simulink model "PathFollowing"  (R2020b)
settings: Solver=FixedStepAuto  StartTime=0.0  StopTime=inf  FixedStep=0.1  RelTol=1e-3
InitFcn:
  | InitParam;
  | SetWaypoints;
StopFcn:
  | plotTrack;
values from neighbouring files (symbols this model uses):
  P0 = [0,0]    [SetWaypoints.m]
  Waypoints = [0 30; 30 30; 30 -30; -30 -30; -30 0; -5 0]    [SetWaypoints.m]
  WPNum = size(Waypoints,1)    [SetWaypoints.m]
  Yaw0 = 70    [SetWaypoints.m]
libraries: vrlib x2, pid_lib x1
settings Model: Creator=53549  LastModifiedBy=53549
settings DataIOCC: ReturnWorkspaceOutputs=off
settings DebuggingCC: ArithmeticOperatorsInVariantConditions=warning
settings SFSimCC: SimUseLocalCustomCode=off  CustomCodeUndefinedFunction=UseInterfaceOnly
settings RTWCC: RTWUseLocalCustomCode=off
settings CodeAppCC: StateflowObjectComments=on

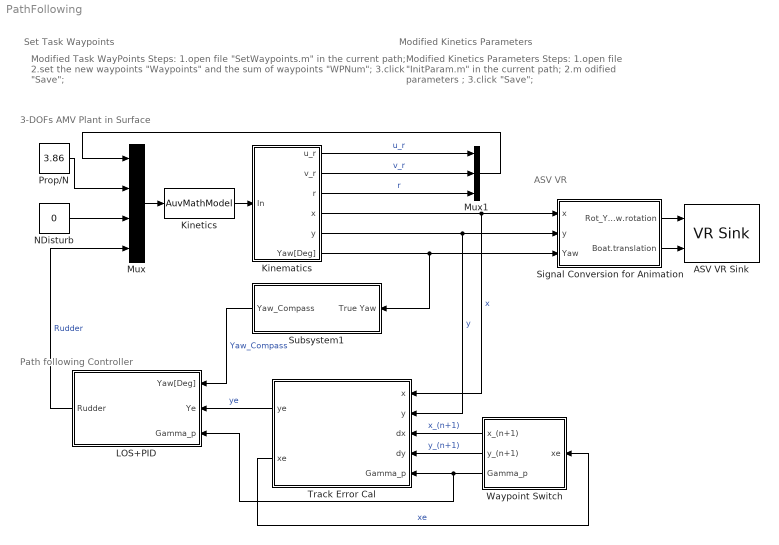
== system PathFollowing ==
  note: ASV VR
  note: Set Task Waypoints
  note: Modified Task WayPoints Steps:
      | 1.open file "SetWaypoints.m" in the current path;
      | 2.set the new waypoints "Waypoints" and the sum of waypoints "WPNum";
      | 3.click "Save";
  note: Path following Controller
  note: 3-DOFs AMV Plant in Surface
  note: Modified Kinetics Parameters
  note: Modified Kinetics Parameters Steps:
      | 1.open file "InitParam.m" in the current path;
      | 2.m odified parameters ;
      | 3.click "Save";
  ASV VR Sink : vrlib/VR Sink  InstantiateOnLoad=on  SampleTime=0.1  ViewEnable=on  RemoteChange=off  RemoteView=off  FieldsWritten=Boat.rotation.4.1.1.double#Boat.translation.3.1.1.double  WorldFileName=ASV.x3d  WorldDescription=ASV Simulation Animation  AutoView=off  VideoDimensions=[]  AllowVariableSize=off  FigureProperties="{'Position', 'Name', 'Viewpoint', 'CameraBound', 'CameraDirection', 'CameraPosition', 'CameraUpVector', 'ZoomFactor', 'Antialiasing', 'Headlight', 'Lighting', 'NavPanel', 'Sound', 'StatusBar', 'Stereo3D', 'Stereo3DCameraOffset', 'Stereo3DHIT', 'ToolBar', 'Textures', 'Transparency', 'Triad', 'Wireframe', 'NavZones', 'NavMode', 'NavSpeed', 'CaptureFileFormat', 'CaptureFileName', 'Record2DCompressMethod', 'Record2DCompressQuality', 'Record2D', 'Record2DFileName', 'Record2DFPS'; [5.0000000000000000e+00   9.2000000000000000e+01   5.7600000000000000e+02   3.5000000000000000e+02], 'ASV Simulation Animation', 'OverView_100m', 'on', [0.0000000000000000e+00   0.0000000000000000e+00  -1.0000000000000000e+00], [0.0000000000000000e+00   0.0000000000000000e+00  -6.0000000000000000e+00], [0.0000000000000000e+00   1.0000000000000000e+00   0.0000000000000000e+00], [1.0000000000000000e+00], 'on', 'on', 'on', 'halfbar', 'on', 'on', 'off', [1.0000000149011612e-01], [0.0000000000000000e+00], 'on', 'on', 'on', 'none', 'off', 'off', 'fly', 'normal', 'tif', '%f_anim_%n.tif', 'auto', [7.5000000000000000e+01], 'off', '%f_anim_%n.avi', 'auto'}"
  "Kinematics " : Subsystem  mask{yawInit=Yaw0, u0=0.4, flowDir=45, flowVel=0.2}
      mask prompts: yawInit "Initial yaw [Deg]"; u0 "Initial velocity [m/s]"; flowDir "Flow direction [Deg]"; flowVel "Flow velocity [m/s]"
      mask DialogControl DescGroupVar Prompt: Kinematics
      mask DialogControl DescTextVar Prompt: Set kinematics information: ASV initial state, flow disturance, etc
      mask DialogControl ParameterGroupVar Prompt: Initial state
      mask DialogControl Container3 Prompt: Flow
  Kinetics : MATLABFcn  MATLABFcn=AuvMathModel  OutputDimensions=3  OutputSignalType=real
  LOS+PID : Subsystem  mask{kp=1, ki=0, kd=1.5, losAlg=ALOS, klos=3, KIlos=0.04}
      mask prompts: losAlg "Guidance Form"
      mask TypeOptions losAlg: LOS | ALOS
      mask DialogControl DescGroupVar Prompt: Path following control
      mask DialogControl DescTextVar Prompt: Please select the guidance law and set the parameters of heading autopilot and line of sight guidance.
      mask DialogControl ParameterGroupVar Prompt: Heading  Autopilot
      mask DialogControl Container3 Prompt: Guidance
  Mux : Mux
  Mux1 : Mux  Inputs=3
  NDisturb : Constant  Value=0
  Prop/N : Constant  Value=3.86
  Signal Conversion for Animation : Subsystem
  Subsystem1 : Subsystem
  Track Error Cal : MATLAB Function  TreatAsAtomicUnit=on
  Waypoint Switch : Subsystem  mask{WP=Waypoints, WPNum=WPNum}
      mask prompts: WP "Waypoints"; WPNum "Waypoints Sum"
      mask DialogControl DescGroupVar Prompt: Task Waypoints
      mask DialogControl DescTextVar Prompt: Please set waypoints and the sum.
  wires:
  Kinetics/1 -> "Kinematics "/1(In)
  Mux/1 -> Kinetics/1
  "Kinematics "/6(Yaw[Deg]) -> Subsystem1/1(True Yaw), Signal Conversion for Animation/3(Yaw)
  "Kinematics "/1(u_r) -> Mux1/1  "u_r"
  "Kinematics "/2(v_r) -> Mux1/2  "v_r"
  "Kinematics "/3(r) -> Mux1/3  "r"
  Mux1/1 -> Mux/1
  Prop/N/1 -> Mux/2
  "Kinematics "/4(x) -> Track Error Cal/1(x), Signal Conversion for Animation/1(x)  "x"
  "Kinematics "/5(y) -> Track Error Cal/2(y), Signal Conversion for Animation/2(y)  "y"
  LOS+PID/1(Rudder) -> Mux/4  "Rudder"
  NDisturb/1 -> Mux/3
  Track Error Cal/1(ye) -> LOS+PID/2(Ye)  "ye"
  Track Error Cal/2(xe) -> Waypoint Switch/1(xe)  "xe"
  Waypoint Switch/1(x_(n+1)) -> Track Error Cal/3(dx)  "x_(n+1)"
  Waypoint Switch/2(y_(n+1)) -> Track Error Cal/4(dy)  "y_(n+1)"
  Waypoint Switch/3(Gamma_p) -> LOS+PID/3(Gamma_p), Track Error Cal/5(Gamma_p)
  Subsystem1/1(Yaw_Compass) -> LOS+PID/1(Yaw[Deg])  "Yaw_Compass"
  Signal Conversion for Animation/1(Rot_Yaw.rotation) -> ASV VR Sink/1
  Signal Conversion for Animation/2(Boat.translation) -> ASV VR Sink/2

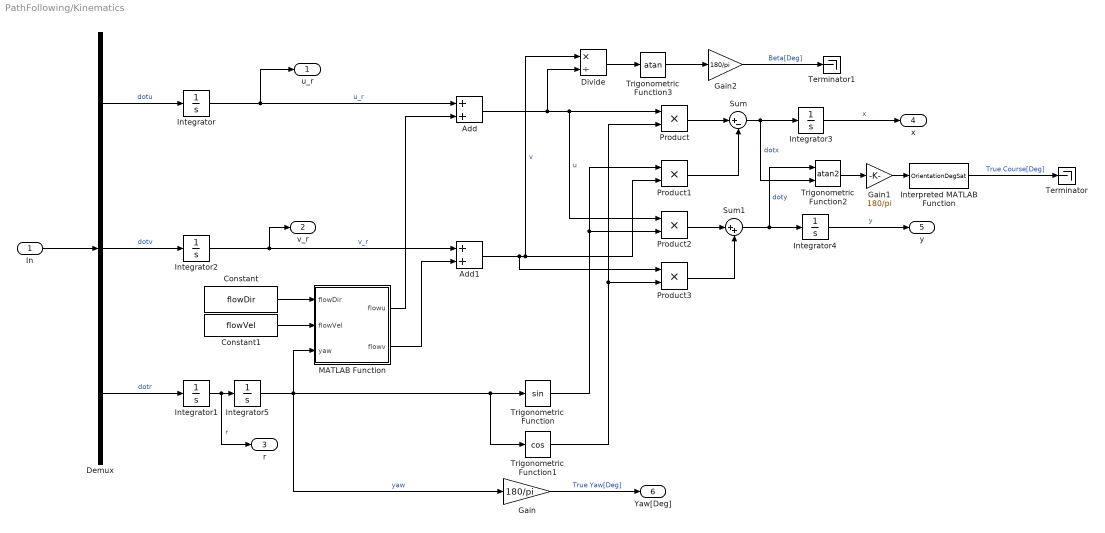
== system PathFollowing/Kinematics  ==
  In : Inport
  Add : Sum
  Add1 : Sum
  Constant : Constant  Value=flowDir
  Constant1 : Constant  Value=flowVel
  Demux : Demux  Outputs=3
  Divide : Product  Inputs=*/
  Gain : Gain  Gain=180/pi
  Gain1 : Gain  Gain=180/pi
  Gain2 : Gain  Gain=180/pi
  Integrator : Integrator  InitialCondition=u0
  Integrator1 : Integrator
  Integrator2 : Integrator
  Integrator3 : Integrator  InitialCondition=P0(1)
  Integrator4 : Integrator  InitialCondition=P0(2)
  Integrator5 : Integrator  InitialCondition=yawInit*pi/180  WrapState=on  WrappedStateUpperValue=6.2832  WrappedStateLowerValue=0
  Interpreted MATLAB Function : MATLABFcn  MATLABFcn=OrientationDegSat
  MATLAB Function : MATLAB Function  TreatAsAtomicUnit=on
  Product{,1..3} (4 alike) : Product
  Sum : Sum  Inputs=|+-
  Sum1 : Sum  Inputs=|++
  Terminator : Terminator
  Terminator1 : Terminator
  Trigonometric Function : Trigonometry
  Trigonometric Function1 : Trigonometry  Operator=cos
  Trigonometric Function2 : Trigonometry  Operator=atan2
  Trigonometric Function3 : Trigonometry  Operator=atan
  u_r : Outport
  v_r : Outport  Port=2
  r : Outport  Port=3
  x : Outport  Port=4
  y : Outport  Port=5
  Yaw[Deg] : Outport  Port=6
  wires:
  Integrator2/1 -> Add1/1, v_r/1  "v_r"
  Integrator3/1 -> x/1  "x"
  Product2/1 -> Sum1/1
  Product1/1 -> Sum/2
  Demux/1 -> Integrator/1  "dotu"
  Demux/2 -> Integrator2/1  "dotv"
  Demux/3 -> Integrator1/1  "dotr"
  Trigonometric Function1/1 -> Product/2, Product3/2
  Product/1 -> Sum/1
  Product3/1 -> Sum1/2
  In/1 -> Demux/1
  Integrator4/1 -> y/1  "y"
  Sum/1 -> Trigonometric Function2/2, Integrator3/1  "dotx"
  Integrator/1 -> Add/1, u_r/1  "u_r"
  Trigonometric Function/1 -> Product1/1, Product2/2
  Sum1/1 -> Trigonometric Function2/1, Integrator4/1  "doty"
  Integrator1/1 -> r/1, Integrator5/1  "r"
  Integrator5/1 -> Gain/1, MATLAB Function/3(yaw), Trigonometric Function1/1, Trigonometric Function/1  "yaw"
  Gain/1 -> Yaw[Deg]/1  "True Yaw[Deg]"
  Constant/1 -> MATLAB Function/1(flowDir)
  Constant1/1 -> MATLAB Function/2(flowVel)
  Add/1 -> Product/1, Product2/1, Divide/2  "u"
  MATLAB Function/1(flowu) -> Add/2
  MATLAB Function/2(flowv) -> Add1/2
  Add1/1 -> Divide/1, Product1/2, Product3/1  "v"
  Trigonometric Function2/1 -> Gain1/1
  Gain1/1 -> Interpreted MATLAB Function/1
  Interpreted MATLAB Function/1 -> Terminator/1  "True Course[Deg]"
  Gain2/1 -> Terminator1/1  "Beta[Deg]"
  Divide/1 -> Trigonometric Function3/1
  Trigonometric Function3/1 -> Gain2/1

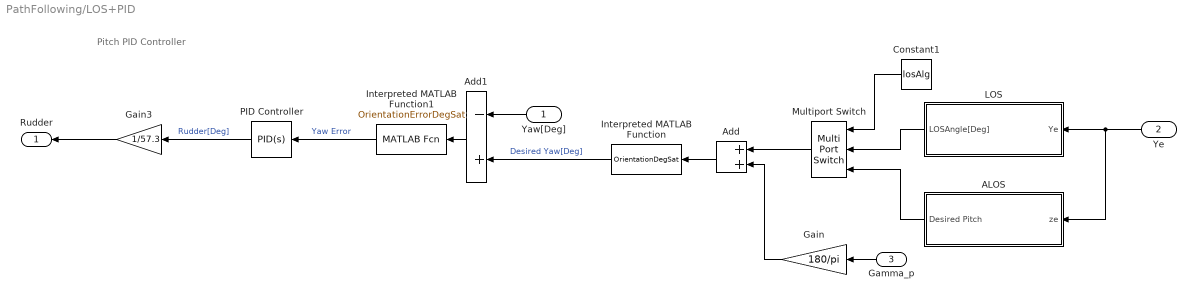
== system PathFollowing/LOS+PID ==
  note: Pitch PID Controller
  Yaw[Deg] : Inport
  Ye : Inport  Port=2
  Gamma_p : Inport  Port=3
  ALOS : Subsystem
  Add : Sum
  Add1 : Sum  Inputs=-+
  Constant1 : Constant  Value=losAlg
  Gain : Gain  Gain=180/pi
  Gain3 : Gain  Gain=1/57.3
  Interpreted MATLAB Function : MATLABFcn  MATLABFcn=OrientationDegSat  OutputDimensions=1
  Interpreted MATLAB Function1 : MATLABFcn  MATLABFcn=OrientationErrorDegSat  OutputDimensions=1
  LOS : Subsystem
  Multiport Switch : MultiPortSwitch  Inputs=2
  PID Controller : pid_lib/PID Controller  Controller=PID  Form=Parallel  TimeDomain=Continuous-time  UseExternalTs=off  SampleTime=-1  IntegratorMethod=Forward Euler  FilterMethod=Forward Euler  ControllerParametersSource=internal  P=kp  I=ki  D=kd  UseFilter=on  N=10  TunerSelectOption=Transfer Function Based (PID Tuner App)  InitialConditionSource=internal  InitialConditionForIntegrator=0  InitialConditionForFilter=0  DifferentiatorICPrevScaledInput=0  ExternalReset=none  TrackingMode=off  Kt=1  LimitOutput=on  SatLimitsSource=internal  UpperSaturationLimit=20  LowerSaturationLimit=-20  LinearizeAsGain=on  AntiWindupMode=none  Kb=1  POutMin=[]  POutMax=[]  IOutMin=[]  IOutMax=[]  DOutMin=[]  DOutMax=[]  NOutMin=[]  NOutMax=[]  SumOutMin=[]  SumOutMax=[]  SaturationOutMin=[]  SaturationOutMax=[]  PParamMin=[]  PParamMax=[]  IParamMin=[]  IParamMax=[]  DParamMin=[]  DParamMax=[]  NParamMin=[]  NParamMax=[]  KbParamMin=[]  KbParamMax=[]  KtParamMin=[]  KtParamMax=[]  KbOutMin=[]  KbOutMax=[]  KtOutMin=[]  KtOutMax=[]  IntegratorOutMin=[]  IntegratorOutMax=[]  FilterOutMin=[]  FilterOutMax=[]  SumI1OutMin=[]  SumI1OutMax=[]  SumI2OutMin=[]  SumI2OutMax=[]  SumI3OutMin=[]  SumI3OutMax=[]  SumI4OutMin=[]  SumI4OutMax=[]  SumDOutMin=[]  SumDOutMax=[]  DifferentiatorOutMin=[]  DifferentiatorOutMax=[]  FilterDiffOutCoefMin=[]  FilterDiffOutCoefMax=[]  ReciprocalOutMin=[]  ReciprocalOutMax=[]  SumDenOutMin=[]  SumDenOutMax=[]  SumNumOutMin=[]  SumNumOutMax=[]  DivideOutMin=[]  DivideOutMax=[]  UdiffTsProdOutMin=[]  UdiffTsProdOutMax=[]  NTsProdOutMin=[]  NTsProdOutMax=[]  UintegralTsProdOutMin=[]  UintegralTsProdOutMax=[]  UngainTsProdOutMin=[]  UngainTsProdOutMax=[]  IntegratorContinuousStateAttributes=''  IntegratorStateMustResolveToSignalObject=off  IntegratorRTWStateStorageClass=Auto  FilterContinuousStateAttributes=''  FilterStateMustResolveToSignalObject=off  FilterRTWStateStorageClass=Auto  ParallelPVariant=InternalParameters  IdealPVariant=Disabled  IVariant=InternalParameters  DVariant=InternalParameters  IntegratorVariant=Continuous  SatVariant=Enabled  AWVariant=Passthrough  PCopyVariant=Disabled  TRVariant=Disabled  FdbkBlocksVariant=Forward  IdealPFdbkVariant=Disabled  SatFdbkVariant=Disabled  DerivativeFilterVariant=ContFilter  NVariant=InternalParameters  NCopyVariant=Disabled  FilterICVariant=InternalICsFilter  IntegratorICVariant=InternalICs  ExternalResetVariant=Disabled  TRSumVariant=Passthrough  SumFdbkVariant=Disabled  SumVariant=Sum_PID  TsampFilterVariant=InternalTs  TsampNgainVariant=Passthrough  TsampIntegralVariant=Passthrough  ExternalSaturationOutDataTypeStr=Inherit: Same as second input
  Rudder : Outport
  wires:
  Gain3/1 -> Rudder/1
  Yaw[Deg]/1 -> Add1/1
  PID Controller/1 -> Gain3/1  "Rudder[Deg]"
  Add1/1 -> Interpreted MATLAB Function1/1
  Interpreted MATLAB Function/1 -> Add1/2  "Desired Yaw[Deg]"
  Ye/1 -> ALOS/1(ze), LOS/1(Ye)
  ALOS/1(Desired Pitch) -> Multiport Switch/3
  LOS/1(LOSAngle[Deg]) -> Multiport Switch/2
  Multiport Switch/1 -> Add/1
  Constant1/1 -> Multiport Switch/1
  Gamma_p/1 -> Gain/1
  Add/1 -> Interpreted MATLAB Function/1
  Gain/1 -> Add/2
  Interpreted MATLAB Function1/1 -> PID Controller/1  "Yaw Error"

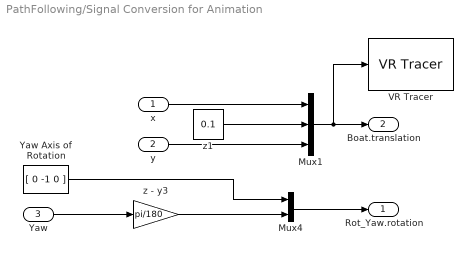
== system PathFollowing/Signal Conversion for Animation ==
  x : Inport
  y : Inport  Port=2
  Yaw : Inport  Port=3
  Mux1 : Mux  Inputs=3
  Mux4 : Mux  Inputs=2
  VR Tracer : vrlib/VR Tracer  VrmlFile=ASV.x3d  MarkerName=None  UseLines=on  UseTriads=off  MarkerScale=[1 1 1]  MarkerColorSelection=Defined as RGB values  MarkerColor=red  rgbval=[1 0 0]  Ts=0.5  ForceViewerOpen=off  ConnectPlane=off  PlaneCoeff=[0 1 0 0]  ConnectPoint=None  PointCoord=[0 0 0]
      settings: SourceProductBaseCode=SL
  Yaw Axis of Rotation : Constant  Value=[ 0 -1 0 ]
  z - y3 : Gain  Gain=pi/180
  z1 : Constant  Value=0.1
  Rot_Yaw.rotation : Outport
  Boat.translation : Outport  Port=2
  wires:
  Yaw Axis of Rotation/1 -> Mux4/1
  Mux1/1 -> VR Tracer/1, Boat.translation/1
  x/1 -> Mux1/1
  Mux4/1 -> Rot_Yaw.rotation/1
  Yaw/1 -> z - y3/1
  z - y3/1 -> Mux4/2
  y/1 -> Mux1/3
  z1/1 -> Mux1/2

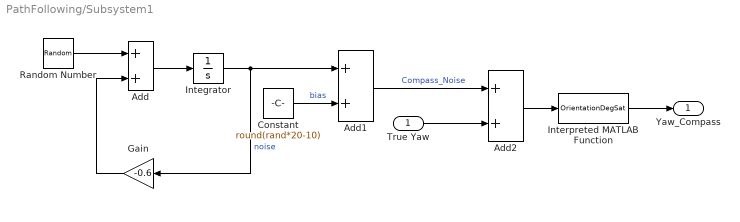
== system PathFollowing/Subsystem1 ==
  True Yaw : Inport
  Add : Sum
  Add1 : Sum
  Add2 : Sum
  Constant : Constant  Value=round(rand*20-10)
  Gain : Gain  Gain=-0.6
  Integrator : Integrator
  Interpreted MATLAB Function : MATLABFcn  MATLABFcn=OrientationDegSat
  Random Number : RandomNumber  Variance=0.2  Seed=round(rand*20)  SampleTime=10
  Yaw_Compass : Outport
  wires:
  Constant/1 -> Add1/2  "bias"
  Random Number/1 -> Add/1
  Integrator/1 -> Add1/1, Gain/1  "noise"
  Gain/1 -> Add/2
  Add/1 -> Integrator/1
  Add1/1 -> Add2/1  "Compass_Noise"
  True Yaw/1 -> Add2/2
  Interpreted MATLAB Function/1 -> Yaw_Compass/1
  Add2/1 -> Interpreted MATLAB Function/1

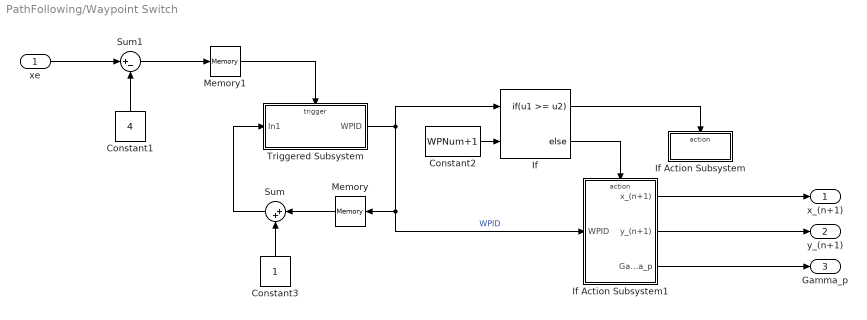
== system PathFollowing/Waypoint Switch ==
  xe : Inport
  Constant1 : Constant  Value=4
  Constant2 : Constant  Value=WPNum+1
  Constant3 : Constant
  If : If  NumInputs=2  IfExpression=u1 >= u2
  If Action Subsystem : Subsystem  TreatAsAtomicUnit=on
  If Action Subsystem1 : Subsystem  TreatAsAtomicUnit=on
  Memory : Memory  InitialCondition=1  InheritSampleTime=on
  Memory1 : Memory  InitialCondition=5  InheritSampleTime=on
  Sum : Sum  Inputs=|++
  Sum1 : Sum  Inputs=|+-
  Triggered Subsystem : Subsystem  TreatAsAtomicUnit=on
  x_(n+1) : Outport
  y_(n+1) : Outport  Port=2
  Gamma_p : Outport  Port=3
  wires:
  If Action Subsystem1/2(y_(n+1)) -> y_(n+1)/1
  Constant2/1 -> If/2
  If Action Subsystem1/3(Gamma_p) -> Gamma_p/1
  Sum1/1 -> Memory1/1
  Memory/1 -> Sum/1
  If/2 -> If Action Subsystem1/Action
  xe/1 -> Sum1/1
  Sum/1 -> Triggered Subsystem/1(In1)
  Constant3/1 -> Sum/2
  If Action Subsystem1/1(x_(n+1)) -> x_(n+1)/1
  Triggered Subsystem/1(WPID) -> If/1, If Action Subsystem1/1(WPID), Memory/1  "WPID"
  Constant1/1 -> Sum1/2
  If/1 -> If Action Subsystem/Action
  Memory1/1 -> Triggered Subsystem/Trigger

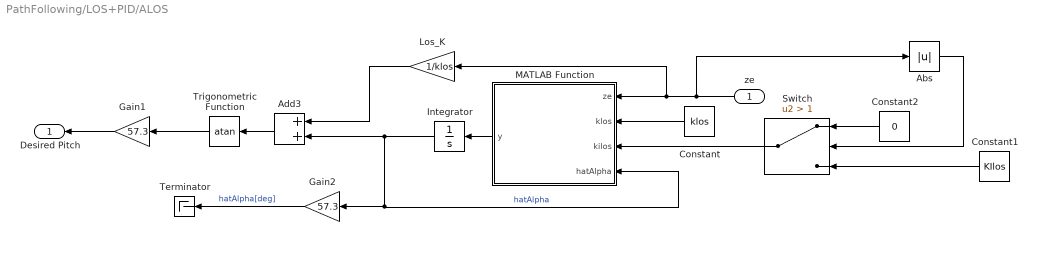
== system PathFollowing/LOS+PID/ALOS ==
  ze : Inport
  Abs : Abs
  Add3 : Sum
  Constant : Constant  Value=klos
  Constant1 : Constant  Value=KIlos
  Constant2 : Constant  Value=0
  Gain1 : Gain  Gain=57.3
  Gain2 : Gain  Gain=57.3
  Integrator : Integrator
  Los_K : Gain  Gain=1/klos
  MATLAB Function : MATLAB Function  TreatAsAtomicUnit=on
  Switch : Switch  Criteria=u2 > Threshold  Threshold=1
  Terminator : Terminator
  Trigonometric Function : Trigonometry  Operator=atan
  Desired Pitch : Outport
  wires:
  Integrator/1 -> MATLAB Function/4(hatAlpha), Gain2/1, Add3/2  "hatAlpha"
  Constant/1 -> MATLAB Function/2(klos)
  MATLAB Function/1(y) -> Integrator/1
  ze/1 -> Abs/1, Los_K/1, MATLAB Function/1(ze)
  Los_K/1 -> Add3/1
  Add3/1 -> Trigonometric Function/1
  Gain1/1 -> Desired Pitch/1
  Trigonometric Function/1 -> Gain1/1
  Gain2/1 -> Terminator/1  "hatAlpha[deg]"
  Switch/1 -> MATLAB Function/3(kilos)
  Constant1/1 -> Switch/3
  Abs/1 -> Switch/2
  Constant2/1 -> Switch/1

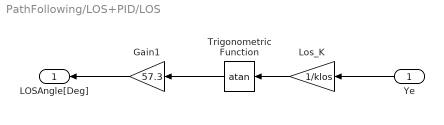
== system PathFollowing/LOS+PID/LOS ==
  Ye : Inport
  Gain1 : Gain  Gain=57.3
  Los_K : Gain  Gain=1/klos
  Trigonometric Function : Trigonometry  Operator=atan
  LOSAngle[Deg] : Outport
  wires:
  Los_K/1 -> Trigonometric Function/1
  Ye/1 -> Los_K/1
  Gain1/1 -> LOSAngle[Deg]/1
  Trigonometric Function/1 -> Gain1/1

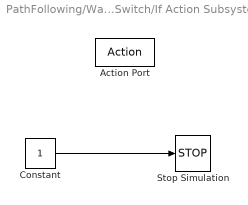
== system PathFollowing/Waypoint Switch/If Action Subsystem ==
  Action Port : ActionPort  ActionPortLabel=if(u1 >= u2)
  Constant : Constant
  Stop Simulation : Stop
  wires:
  Constant/1 -> Stop Simulation/1

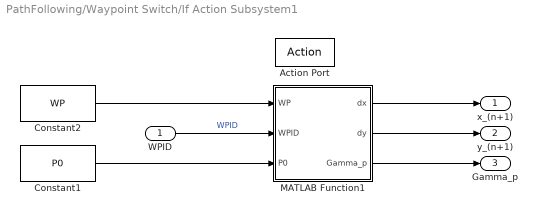
== system PathFollowing/Waypoint Switch/If Action Subsystem1 ==
  WPID : Inport
  Action Port : ActionPort  ActionPortLabel=else
  Constant1 : Constant  Value=P0
  Constant2 : Constant  Value=WP
  MATLAB Function1 : MATLAB Function  TreatAsAtomicUnit=on
  x_(n+1) : Outport
  y_(n+1) : Outport  Port=2
  Gamma_p : Outport  Port=3
  wires:
  MATLAB Function1/3(Gamma_p) -> Gamma_p/1
  MATLAB Function1/1(dx) -> x_(n+1)/1
  MATLAB Function1/2(dy) -> y_(n+1)/1
  Constant2/1 -> MATLAB Function1/1(WP)
  WPID/1 -> MATLAB Function1/2(WPID)  "WPID"
  Constant1/1 -> MATLAB Function1/3(P0)

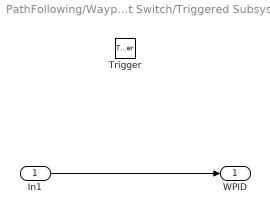
== system PathFollowing/Waypoint Switch/Triggered Subsystem ==
  In1 : Inport
  Trigger : TriggerPort  TriggerType=falling  VariantControl=Variant
  WPID : Outport  InitialOutput=1
  wires:
  In1/1 -> WPID/1

== matlab function PathFollowing/Waypoint Switch/If Action Subsystem1/MATLAB Function1 ==
  data: dx output; WP input; dy output; WPID input; Gamma_p output; P0 input
function [dx,dy,Gamma_p] = fcn(WP,WPID,P0)
dx = WP(WPID,1);
dy = WP(WPID,2);
if WPID == 1
    Gamma_p = atan2(dy-P0(2),dx-P0(1));
else
    Gamma_p = atan2(dy-WP(WPID-1,2),dx-WP(WPID-1,1));
end
if Gamma_p<0
    Gamma_p = Gamma_p + 2*pi;
end

== matlab function PathFollowing/Track Error Cal ==
  data: ye output; x input; xe output; y input; dx input; dy input; Gamma_p input
function [ye,xe] = fcn(x,y,dx,dy,Gamma_p)
xe = (dx-x)*cos(Gamma_p)+(dy-y)*sin(Gamma_p);
ye = -(dx-x)*sin(Gamma_p)+(dy-y)*cos(Gamma_p);

== matlab function PathFollowing/LOS+PID/ALOS/MATLAB Function ==
  data: ze input; y output; klos input; kilos input; hatAlpha input
function y = fcn(ze,klos,kilos,hatAlpha)
y =1.45*ze*klos*kilos/sqrt(klos*klos+(ze+klos*hatAlpha)*(ze+klos*hatAlpha));

== matlab function PathFollowing/Kinematics /MATLAB Function ==
  data: flowDir input; flowu output; flowVel input; yaw input; flowv output
function [flowu,flowv] = fcn(flowDir,flowVel,yaw)
dAngle = flowDir - yaw;
if dAngle > 2*pi
    dAngle = dAngle-2*pi;
elseif dAngle<0
    dAngle = dAngle+2*pi;
end
flowu = flowVel*cos(dAngle);
flowv = flowVel*sin(dAngle);
